simulink model "Backup"  (R2018a)
settings: Solver=VariableStepAuto  StartTime=0.0  StopTime=3  RelTol=1e-3
libraries: powerlib x15, simulink x4, rectifier_leg x3, inverter_leg x3, powerlib_meascontrol x1
settings Model: Creator=elasfory  LastModifiedBy=AL-MOSTAFA

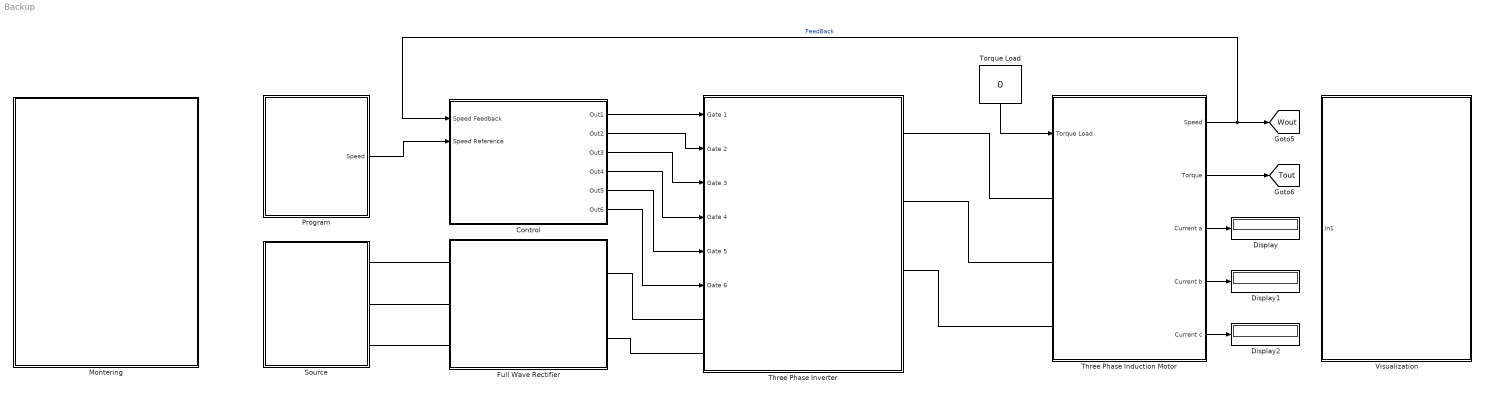
== system Backup ==
  Control : Subsystem
  Display : Display
  Display1 : Display
  Display2 : Display
  Full Wave Rectifier : Subsystem
  Montering : Subsystem
  Program : Subsystem
  Source : Subsystem
  Three Phase Induction Motor : Subsystem
  Three Phase Inverter : Subsystem
  Torque Load : Constant  Value=0
  Visualization : Subsystem
  tag scope: Tout=global, Wout=global
  wires:
  Control/6(Out6) -> Three Phase Inverter/6(Gate 6)
  Control/5(Out5) -> Three Phase Inverter/5(Gate 5)
  Control/4(Out4) -> Three Phase Inverter/4(Gate 4)
  Control/3(Out3) -> Three Phase Inverter/3(Gate 3)
  Control/2(Out2) -> Three Phase Inverter/2(Gate 2)
  Control/1(Out1) -> Three Phase Inverter/1(Gate 1)
  Three Phase Induction Motor/1(Speed) -> Control/1(Speed Feedback), [Wout]  "FeedBack"
  Three Phase Induction Motor/2(Torque) -> [Tout]
  Torque Load/1 -> Three Phase Induction Motor/1(Torque Load)
  Program/1(Speed) -> Control/2(Speed Reference)
  Three Phase Induction Motor/3(Current a) -> Display/1
  Three Phase Induction Motor/4(Current b) -> Display1/1
  Three Phase Induction Motor/5(Current c) -> Display2/1
  connections:
  Three Phase Inverter/LConn1 -- Full Wave Rectifier/RConn1
  Full Wave Rectifier/RConn2 -- Three Phase Inverter/LConn2
  Source/RConn1 -- Full Wave Rectifier/LConn1
  Source/RConn2 -- Full Wave Rectifier/LConn2
  Source/RConn3 -- Full Wave Rectifier/LConn3
  Three Phase Inverter/RConn1 -- Three Phase Induction Motor/LConn1
  Three Phase Inverter/RConn2 -- Three Phase Induction Motor/LConn2
  Three Phase Inverter/RConn3 -- Three Phase Induction Motor/LConn3

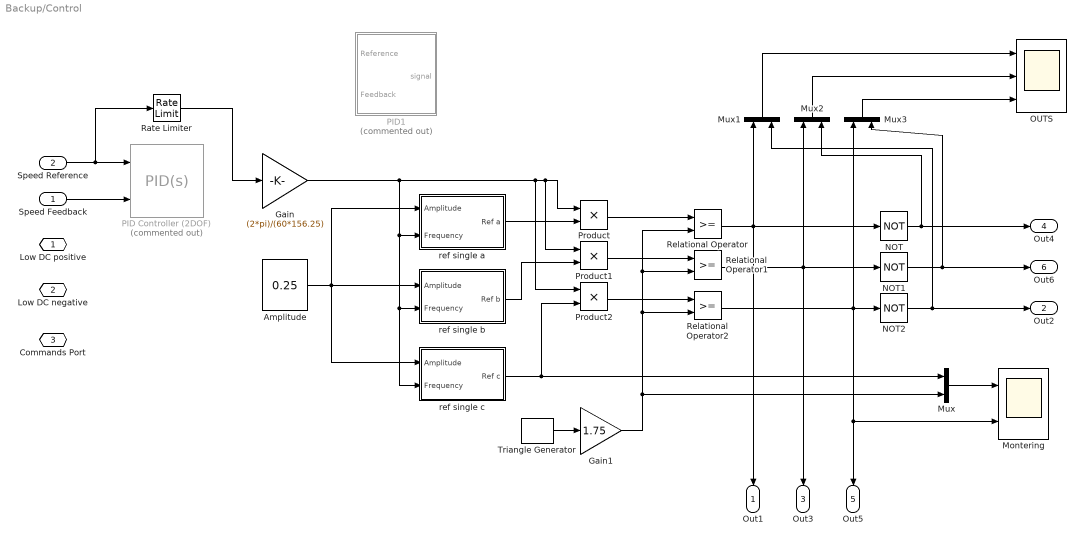
== system Backup/Control ==
  Speed Feedback : Inport
  Speed Reference : Inport  Port=2
  Amplitude : Constant  Value=0.25
  Gain : Gain  Gain=(2*pi)/(60*156.25)
  Gain1 : Gain  Gain=1.75
  Montering : Scope  NumInputPorts=2
  Mux{,1..3} (4 alike) : Mux  Inputs=2
  NOT : Logic  Operator=NOT  IconShape=distinctive  AllPortsSameDT=off  OutDataTypeStr=boolean
  NOT1 : Logic  Operator=NOT  IconShape=distinctive  AllPortsSameDT=off  OutDataTypeStr=boolean
  NOT2 : Logic  Operator=NOT  IconShape=distinctive  AllPortsSameDT=off  OutDataTypeStr=boolean
  OUTS : Scope  NumInputPorts=3
  PID Controller (2DOF) : simulink/Continuous/PID Controller (2DOF)  Commented=on  Controller=PID  TimeDomain=Continuous-time  SampleTime=-1  IntegratorMethod=Forward Euler  FilterMethod=Forward Euler  Form=Parallel  UseFilter=on  ControllerParametersSource=internal  P=1  I=0.1  D=0  N=100  b=1  c=1  InitialConditionSource=internal  InitialConditionForIntegrator=0  InitialConditionForFilter=0  ExternalReset=none  LimitOutput=off  UpperSaturationLimit=inf  LowerSaturationLimit=-inf  LinearizeAsGain=on  AntiWindupMode=none  Kb=1  TrackingMode=off  Kt=1  PParamMin=[]  PParamMax=[]  IParamMin=[]  IParamMax=[]  DParamMin=[]  DParamMax=[]  NParamMin=[]  NParamMax=[]  bParamMin=[]  bParamMax=[]  cParamMin=[]  cParamMax=[]  KbParamMin=[]  KbParamMax=[]  KtParamMin=[]  KtParamMax=[]  POutMin=[]  POutMax=[]  IOutMin=[]  IOutMax=[]  DOutMin=[]  DOutMax=[]  NOutMin=[]  NOutMax=[]  bOutMin=[]  bOutMax=[]  cOutMin=[]  cOutMax=[]  KbOutMin=[]  KbOutMax=[]  KtOutMin=[]  KtOutMax=[]  IntegratorOutMin=[]  IntegratorOutMax=[]  FilterOutMin=[]  FilterOutMax=[]  SumOutMin=[]  SumOutMax=[]  Sum1OutMin=[]  Sum1OutMax=[]  Sum2OutMin=[]  Sum2OutMax=[]  Sum3OutMin=[]  Sum3OutMax=[]  SumI1OutMin=[]  SumI1OutMax=[]  SumI2OutMin=[]  SumI2OutMax=[]  SumI3OutMin=[]  SumI3OutMax=[]  SumDOutMin=[]  SumDOutMax=[]  SaturationOutMin=[]  SaturationOutMax=[]  IntegratorContinuousStateAttributes=''  IntegratorStateMustResolveToSignalObject=off  IntegratorRTWStateStorageClass=Auto  FilterContinuousStateAttributes=''  FilterStateMustResolveToSignalObject=off  FilterRTWStateStorageClass=Auto  DifferentiatorICPrevScaledInput=0  DifferentiatorOutMin=[]  DifferentiatorOutMax=[]  FilterDiffOutCoefMin=[]  FilterDiffOutCoefMax=[]  SumDenOutMin=[]  SumDenOutMax=[]  SumNumOutMin=[]  SumNumOutMax=[]  ReciprocalOutMin=[]  ReciprocalOutMax=[]  DivideOutMin=[]  DivideOutMax=[]  TunerSelectOption=Transfer Function Based (PID Tuner App)
  PID1 : Subsystem  Commented=on
  Product : Product
  Product1 : Product
  Product2 : Product
  Rate Limiter : RateLimiter  RisingSlewLimit=100  SampleTimeMode=inherited
  Relational Operator : RelationalOperator  OutDataTypeStr=boolean  RndMeth=Simplest
  Relational Operator1 : RelationalOperator  OutDataTypeStr=boolean  RndMeth=Simplest
  Relational Operator2 : RelationalOperator  OutDataTypeStr=boolean  RndMeth=Simplest
  Triangle Generator : powerlib_meascontrol/Pulse & Signal Generators/Triangle Generator  Freq=1e4  Phase=90  Ts=0
  ref single a : Subsystem
  ref single b : Subsystem
  ref single c : Subsystem
  Low DC positive : PMIOPort  Side=Left
  Low DC negative : PMIOPort  Port=2  Side=Left
  Commands Port : PMIOPort  Port=3  Side=Left
  Out1 : Outport
  Out2 : Outport  Port=2
  Out3 : Outport  Port=3
  Out4 : Outport  Port=4
  Out5 : Outport  Port=5
  Out6 : Outport  Port=6
  wires:
  Relational Operator/1 -> Mux1/1, NOT/1, Out1/1
  Relational Operator1/1 -> Mux2/1, Out3/1, NOT1/1
  Relational Operator2/1 -> Mux3/1, Montering/2, Out5/1, NOT2/1
  Triangle Generator/1 -> Gain1/1
  NOT/1 -> Mux2/2, Out4/1
  NOT1/1 -> Mux3/2, Out6/1
  NOT2/1 -> Mux1/2, Out2/1
  ref single a/1(Ref a) -> Product/2
  ref single b/1(Ref b) -> Product1/2
  ref single c/1(Ref c) -> Product2/2, Mux/1
  Gain/1 -> ref single c/2(Frequency), ref single b/2(Frequency), ref single a/2(Frequency), Product2/1, Product/1, Product1/1
  Product/1 -> Relational Operator/1
  Product1/1 -> Relational Operator1/1
  Product2/1 -> Relational Operator2/1
  Amplitude/1 -> ref single a/1(Amplitude), ref single c/1(Amplitude), ref single b/1(Amplitude)
  Gain1/1 -> Relational Operator2/2, Relational Operator1/2, Relational Operator/2, Mux/2
  Mux/1 -> Montering/1
  Speed Reference/1 -> Rate Limiter/1, PID Controller (2DOF)/1
  Speed Feedback/1 -> PID Controller (2DOF)/2
  Rate Limiter/1 -> Gain/1
  Mux1/1 -> OUTS/1
  Mux2/1 -> OUTS/2
  Mux3/1 -> OUTS/3

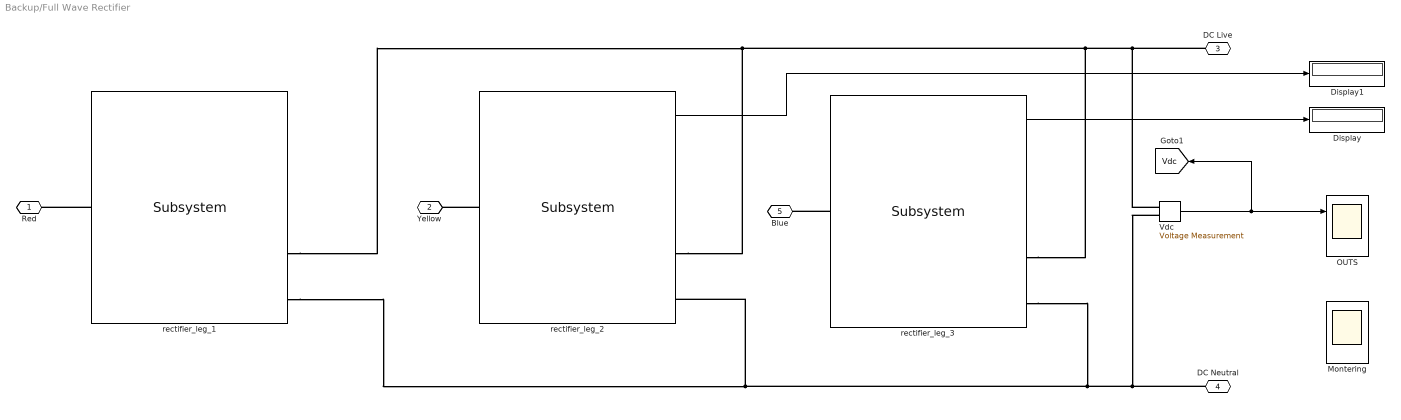
== system Backup/Full Wave Rectifier ==
  Display : Display
  Display1 : Display
  Montering : Scope  NumInputPorts=4
  OUTS : Scope  NumInputPorts=2
  Vdc : powerlib/Measurements/Voltage Measurement  PhasorSimulation=off  OutputType=Complex  PSBequivalent=0
  rectifier_leg_1 : rectifier_leg/Subsystem
  rectifier_leg_2 : rectifier_leg/Subsystem
  rectifier_leg_3 : rectifier_leg/Subsystem
  Red : PMIOPort  Side=Left
  Yellow : PMIOPort  Port=2  Side=Left
  DC Live : PMIOPort  Port=3  Side=Right
  DC Neutral : PMIOPort  Port=4  Side=Right
  Blue : PMIOPort  Port=5  Side=Left
  tag scope: Vdc=global
  wires:
  Vdc/1 -> [Vdc], OUTS/1
  rectifier_leg_3/1 -> Display/1
  rectifier_leg_2/1 -> Display1/1
  connections:
  DC Live/RConn1 -- Vdc/LConn1 -- rectifier_leg_1/RConn1 -- rectifier_leg_2/RConn1 -- rectifier_leg_3/RConn1
  rectifier_leg_1/LConn1 -- Red/RConn1
  rectifier_leg_2/LConn1 -- Yellow/RConn1
  rectifier_leg_3/LConn1 -- Blue/RConn1
  rectifier_leg_3/RConn2 -- DC Neutral/RConn1 -- Vdc/LConn2 -- rectifier_leg_2/RConn2 -- rectifier_leg_1/RConn2

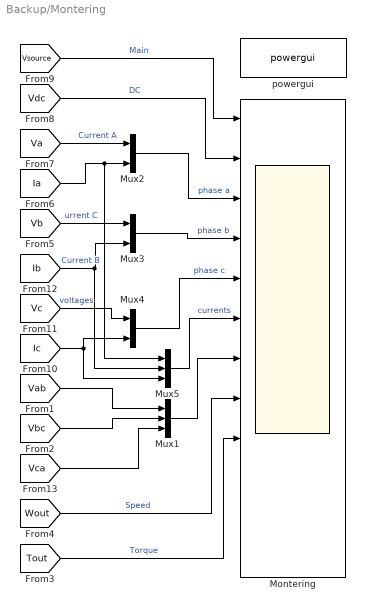
== system Backup/Montering ==
  Montering : Scope  NumInputPorts=12
  Mux1 : Mux  Inputs=3
  Mux2 : Mux  Inputs=2
  Mux3 : Mux  Inputs=2
  Mux4 : Mux  Inputs=2
  Mux5 : Mux  Inputs=3
  powergui : powerlib/powergui  Priority=1  SimulationMode=Continuous  SampleTime=50e-6  frequency=60  Iterations=50  frequencyindice=0  Pbase=100e6  ErrMax=1e-4  UnitsV=kV  UnitsW=MW  buscounter=0  FunctionMessages=off  echomessages=off  EnableUseOfTLC=off  CurrentSourceSwitches=off  DisableSnubberDevices=off  DisableRonSwitches=off  DisableVfSwitches=off  DisplayEquations=off  SolverType=Tustin/Backward Euler (TBE)  Interpol=off  ExternalGateDelay=off  methode=off  Ts=100  x0status=blocks  SPID=on  SwTol=0  HookPort=off  RestoreLinks=warning  ResistiveCurrentMeasurement=off  Frange=[0:2:500]  Ylog=off  Xlog=on  ShowGrid=off  save=off  variable=ZData  structure=0  ZoomFFT=off  StartTime=0.0  cycles=1  DisplayStyle=1  fundamental=60  FreqAxis=off  MaxFrequency=1000  frequencyindicesteady=1  RmsSteady=1  display=off
  wires:
  Mux5/1 -> Montering/6  "currents"
  [Vc] -> Mux4/1  "voltages"
  [Tout] -> Montering/9  "Torque"
  [Wout] -> Montering/8  "Speed"
  [Ic] -> Mux5/3, Mux4/2
  [Vdc] -> Montering/2  "DC"
  [Vb] -> Mux3/1  "urrent C"
  [Vbc] -> Mux1/2
  Mux1/1 -> Montering/7
  [Va] -> Mux2/1  "Current A"
  [Ib] -> Mux5/2, Mux3/2
  [Vca] -> Mux1/3
  [Vab] -> Mux1/1
  Mux3/1 -> Montering/4  "phase b"
  Mux2/1 -> Montering/3  "phase a"
  Mux4/1 -> Montering/5  "phase c"
  [Ia] -> Mux5/1, Mux2/2  "Current B"
  [Vsource] -> Montering/1  "Main"

== system Backup/Program ==
  RPM : Constant  Value=1400
  Speed : Outport
  wires:
  RPM/1 -> Speed/1

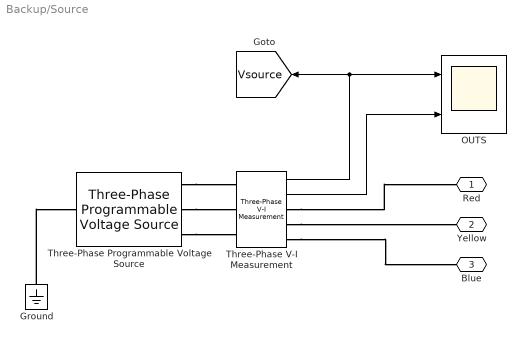
== system Backup/Source ==
  Ground : powerlib/Elements/Ground  LConnTagsString=a
  OUTS : Scope  NumInputPorts=2
  Three-Phase Programmable Voltage Source : powerlib/Electrical Sources/Three-Phase Programmable Voltage Source  PositiveSequence="[380  0 50]"  VariationEntity=None  VariationType=Table of time-amplitude pairs  VariationTypeAlt=Step  VariationStep=0.5  VariationRate=10  VariationMagnitude=0.3  VariationFrequency=2  VariationTiming=[1 2]  VariationPhaseA=off  Amplitudes=[1 0.8 1.2 1.0]  TimeValues=[0 0.1 0.15 0.2]  HarmonicGeneration=off  HarmonicA=[3 0.2 -25 0]  HarmonicB=[2 0.15 35 2]  Timing="[0.05  3]"  BusType=swing  Pref=0  Qref=0  Qmin=-inf  Qmax=inf
  Three-Phase V-I Measurement : powerlib/Measurements/Three-Phase V-I Measurement  VoltageMeasurement=phase-to-ground  SetLabelV=off  LabelV=Vabc  Vpu=off  VpuLL=off  CurrentMeasurement=yes  SetLabelI=off  LabelI=Iabc  Ipu=off  Pbase=100e6  Vbase=500e3  OutputType=Complex  PhasorSimulation=off  PSBequivalent=0
  Red : PMIOPort  Side=Right
  Yellow : PMIOPort  Port=2  Side=Right
  Blue : PMIOPort  Port=3  Side=Right
  tag scope: Vsource=global
  wires:
  Three-Phase V-I Measurement/1 -> [Vsource], OUTS/1
  Three-Phase V-I Measurement/2 -> OUTS/2
  connections:
  Three-Phase V-I Measurement/RConn3 -- Blue/RConn1
  Three-Phase V-I Measurement/RConn1 -- Red/RConn1
  Three-Phase V-I Measurement/RConn2 -- Yellow/RConn1
  Three-Phase Programmable Voltage Source/RConn1 -- Three-Phase V-I Measurement/LConn1
  Three-Phase Programmable Voltage Source/RConn2 -- Three-Phase V-I Measurement/LConn2
  Three-Phase Programmable Voltage Source/RConn3 -- Three-Phase V-I Measurement/LConn3
  Ground/LConn1 -- Three-Phase Programmable Voltage Source/LConn1

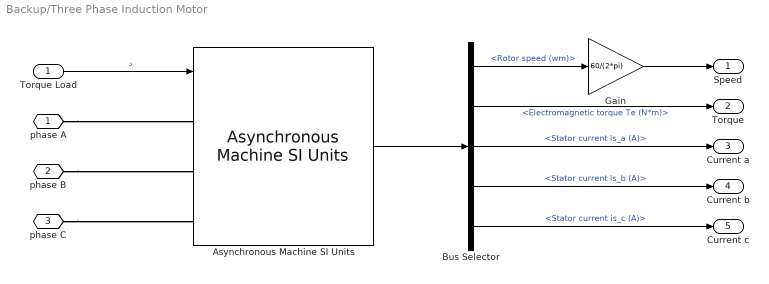
== system Backup/Three Phase Induction Motor ==
  Torque Load : Inport
  Asynchronous Machine SI Units : powerlib/Machines/Asynchronous Machine SI Units  RotorType=Squirrel-cage  PresetModel="15:  5.4 HP (4KW)   400 V  50Hz 1430 RPM"  MechanicalLoad=Torque Tm  ShowDetailedParameters=on  ReferenceFrame=Stationary  Units=SI  MeasurementBus=off  NominalParameters=[4000 400 50]  Stator=[1.405 0.005839]  Rotor=[1.395 0.005839]  Cage1=[0.4155 0.002066]  Cage2=[0.4168 0.0003495]  Lm=0.1722  Mechanical=[0.0131 0.002985 2]  PolePairs=2  InitialConditions=[1 0 0 0 0 0 0 0]  SimulateSaturation=off  Saturation=[14.03593122, 27.81365428, 53.79336849, 72.68890987, 97.98006896, 148.6815601, 215.7428561, 302.9841135, 428.7778367 ; 230, 322, 414, 460, 506, 552, 598, 644, 690]  LoadFlowParameters=1492000  TsPowergui=0  TsBlock=-1  IterativeModel=Trapezoidal non iterative  IterativeDiscreteModel=Trapezoidal non iterative  Pmec=1.492e+006
  Bus Selector : BusSelector  OutputSignals=Mechanical.Rotor speed (wm),Mechanical.Electromagnetic torque Te (N*m),Stator measurements.Stator current is_a (A),Stator measurements.Stator current is_b (A),Stator measurements.Stator current is_c (A)
  Gain : Gain  Gain=60/(2*pi)
  phase A : PMIOPort  Side=Left
  phase B : PMIOPort  Port=2  Side=Left
  phase C : PMIOPort  Port=3  Side=Left
  Speed : Outport
  Torque : Outport  Port=2
  Current a : Outport  Port=3
  Current b : Outport  Port=4
  Current c : Outport  Port=5
  wires:
  Asynchronous Machine SI Units/1 -> Bus Selector/1
  Bus Selector/2 -> Torque/1  "<Electromagnetic torque Te (N*m)>"
  Torque Load/1 -> Asynchronous Machine SI Units/1  "د"
  Bus Selector/3 -> Current a/1  "<Stator current is_a (A)>"
  Bus Selector/4 -> Current b/1  "<Stator current is_b (A)>"
  Bus Selector/5 -> Current c/1  "<Stator current is_c (A)>"
  Bus Selector/1 -> Gain/1  "<Rotor speed (wm)>"
  Gain/1 -> Speed/1
  connections:
  phase B/RConn1 -- Asynchronous Machine SI Units/LConn2
  phase A/RConn1 -- Asynchronous Machine SI Units/LConn1
  phase C/RConn1 -- Asynchronous Machine SI Units/LConn3

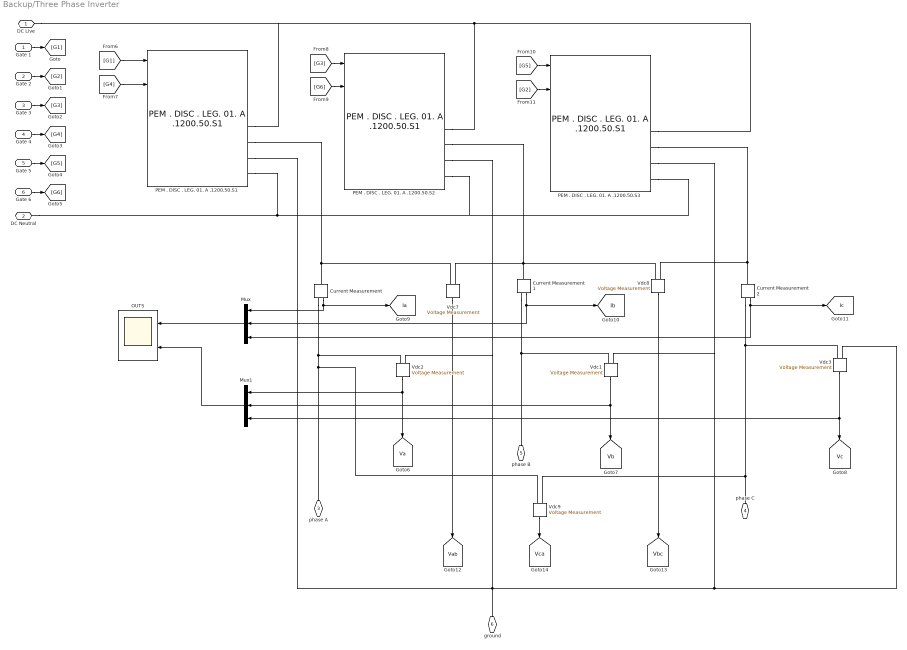
== system Backup/Three Phase Inverter ==
  Gate 1 : Inport
  Gate 2 : Inport  Port=2
  Gate 3 : Inport  Port=3
  Gate 4 : Inport  Port=4
  Gate 5 : Inport  Port=5
  Gate 6 : Inport  Port=6
  Current Measurement : powerlib/Measurements/Current Measurement  PhasorSimulation=off  OutputType=Complex  PSBequivalent=0
  Current Measurement1 : powerlib/Measurements/Current Measurement  PhasorSimulation=off  OutputType=Complex  PSBequivalent=0
  Current Measurement2 : powerlib/Measurements/Current Measurement  PhasorSimulation=off  OutputType=Complex  PSBequivalent=0
  Mux : Mux  Inputs=3
  Mux1 : Mux  Inputs=3
  OUTS : Scope  NumInputPorts=2
  PEM . DISC . LEG. 01. A .1200.50.S1 : inverter_leg/PEM . DISC . LEG. 01. A .1200.50.S1
  PEM . DISC . LEG. 01. A .1200.50.S2 : inverter_leg/PEM . DISC . LEG. 01. A .1200.50.S1
  PEM . DISC . LEG. 01. A .1200.50.S3 : inverter_leg/PEM . DISC . LEG. 01. A .1200.50.S1
  Vdc{1..3,7..9} (6 alike) : powerlib/Measurements/Voltage Measurement  PhasorSimulation=off  OutputType=Complex  PSBequivalent=0
  DC Live : PMIOPort  Side=Left
  DC Neutral : PMIOPort  Port=2  Side=Left
  phase A : PMIOPort  Port=3  Side=Right
  phase C : PMIOPort  Port=4  Side=Right
  phase B : PMIOPort  Port=5  Side=Right
  ground : PMIOPort  Port=6  Side=Right
  tag scope: Ia=global, Ib=global, Ic=global, Va=global, Vab=global, Vb=global, Vbc=global, Vc=global, Vca=global
  wires:
  Gate 1/1 -> [G1]
  Gate 2/1 -> [G2]
  Gate 3/1 -> [G3]
  Gate 4/1 -> [G4]
  Gate 5/1 -> [G5]
  Gate 6/1 -> [G6]
  [G4] -> PEM . DISC . LEG. 01. A .1200.50.S1/2
  [G1] -> PEM . DISC . LEG. 01. A .1200.50.S1/1
  [G6] -> PEM . DISC . LEG. 01. A .1200.50.S2/2
  [G3] -> PEM . DISC . LEG. 01. A .1200.50.S2/1
  [G5] -> PEM . DISC . LEG. 01. A .1200.50.S3/1
  [G2] -> PEM . DISC . LEG. 01. A .1200.50.S3/2
  Current Measurement/1 -> [Ia], Mux/1
  Current Measurement1/1 -> Mux/2, [Ib]
  Current Measurement2/1 -> Mux/3, [Ic]
  Vdc2/1 -> [Va], Mux1/1
  Vdc1/1 -> Mux1/2, [Vb]
  Vdc3/1 -> Mux1/3, [Vc]
  Vdc9/1 -> [Vca]
  Vdc7/1 -> [Vab]
  Vdc8/1 -> [Vbc]
  Mux/1 -> OUTS/1
  Mux1/1 -> OUTS/2
  connections:
  PEM . DISC . LEG. 01. A .1200.50.S1/RConn1 -- DC Live/RConn1 -- PEM . DISC . LEG. 01. A .1200.50.S3/RConn1 -- PEM . DISC . LEG. 01. A .1200.50.S2/RConn1
  PEM . DISC . LEG. 01. A .1200.50.S3/RConn4 -- PEM . DISC . LEG. 01. A .1200.50.S2/RConn4 -- PEM . DISC . LEG. 01. A .1200.50.S1/RConn4 -- DC Neutral/RConn1
  ground/RConn1 -- PEM . DISC . LEG. 01. A .1200.50.S1/RConn3 -- PEM . DISC . LEG. 01. A .1200.50.S3/RConn3 -- Vdc1/LConn2 -- Vdc3/LConn2 -- PEM . DISC . LEG. 01. A .1200.50.S2/RConn3 -- Vdc2/LConn2
  Current Measurement/LConn1 -- PEM . DISC . LEG. 01. A .1200.50.S1/RConn2 -- Vdc7/LConn1
  Current Measurement/RConn1 -- Vdc2/LConn1 -- Vdc9/LConn2 -- phase A/RConn1
  Current Measurement1/RConn1 -- Vdc1/LConn1 -- phase B/RConn1
  Current Measurement1/LConn1 -- PEM . DISC . LEG. 01. A .1200.50.S2/RConn2 -- Vdc8/LConn1 -- Vdc7/LConn2
  Current Measurement2/RConn1 -- Vdc3/LConn1 -- Vdc9/LConn1 -- phase C/RConn1
  Current Measurement2/LConn1 -- PEM . DISC . LEG. 01. A .1200.50.S3/RConn2 -- Vdc8/LConn2

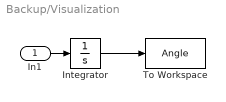
== system Backup/Visualization ==
  In1 : Inport
  Integrator : Integrator
  To Workspace : ToWorkspace  VariableName=Angle  SaveFormat=Timeseries  SampleTime=0.001
      settings: MaxDataPoints=10
  wires:
  Integrator/1 -> To Workspace/1
  In1/1 -> Integrator/1

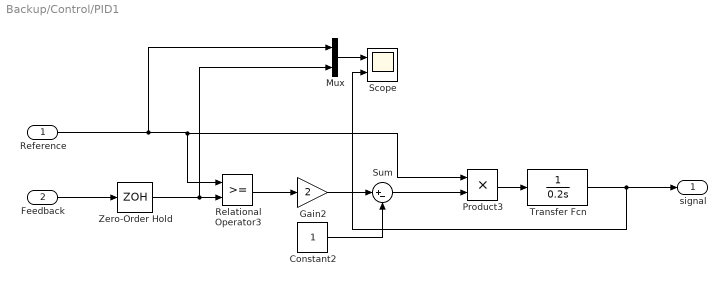
== system Backup/Control/PID1 ==
  Reference : Inport
  Feedback : Inport  Port=2
  Constant2 : Constant
  Gain2 : Gain  Gain=2
  Mux : Mux  Inputs=2
  Product3 : Product
  Relational Operator3 : RelationalOperator  OutDataTypeStr=boolean  RndMeth=Simplest
  Scope : Scope  NumInputPorts=2
  Sum : Sum  Inputs=|+-
  Transfer Fcn : TransferFcn  Denominator=[0.2 0]
  Zero-Order Hold : ZeroOrderHold  SampleTime=1e-2
  signal : Outport
  wires:
  Zero-Order Hold/1 -> Mux/2, Relational Operator3/2
  Relational Operator3/1 -> Gain2/1
  Constant2/1 -> Sum/2
  Sum/1 -> Product3/2
  Gain2/1 -> Sum/1
  Product3/1 -> Transfer Fcn/1
  Reference/1 -> Mux/1, Product3/1, Relational Operator3/1
  Transfer Fcn/1 -> Scope/2, signal/1
  Mux/1 -> Scope/1
  Feedback/1 -> Zero-Order Hold/1

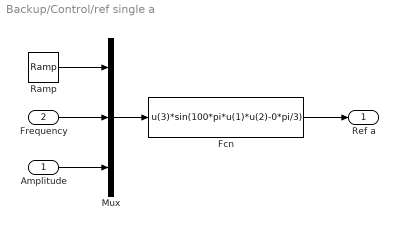
== system Backup/Control/ref single a ==
  Amplitude : Inport
  Frequency : Inport  Port=2
  Fcn : Fcn  Expr=u(3)*sin(100*pi*u(1)*u(2)-0*pi/3)
  Mux : Mux  Inputs=3
  Ramp : simulink/Sources/Ramp  slope=1  start=0  InitialOutput=0
  Ref a : Outport
  wires:
  Mux/1 -> Fcn/1
  Frequency/1 -> Mux/2
  Ramp/1 -> Mux/1
  Fcn/1 -> Ref a/1
  Amplitude/1 -> Mux/3

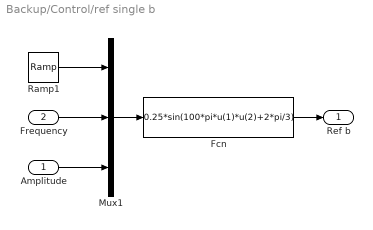
== system Backup/Control/ref single b ==
  Amplitude : Inport
  Frequency : Inport  Port=2
  Fcn : Fcn  Expr=0.25*sin(100*pi*u(1)*u(2)+2*pi/3)
  Mux1 : Mux  Inputs=3
  Ramp1 : simulink/Sources/Ramp  slope=1  start=0  InitialOutput=0
  Ref b : Outport
  wires:
  Fcn/1 -> Ref b/1
  Ramp1/1 -> Mux1/1
  Frequency/1 -> Mux1/2
  Mux1/1 -> Fcn/1
  Amplitude/1 -> Mux1/3

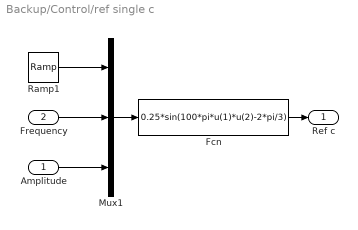
== system Backup/Control/ref single c ==
  Amplitude : Inport
  Frequency : Inport  Port=2
  Fcn : Fcn  Expr=0.25*sin(100*pi*u(1)*u(2)-2*pi/3)
  Mux1 : Mux  Inputs=3
  Ramp1 : simulink/Sources/Ramp  slope=1  start=0  InitialOutput=0
  Ref c : Outport
  wires:
  Fcn/1 -> Ref c/1
  Amplitude/1 -> Mux1/3
  Mux1/1 -> Fcn/1
  Frequency/1 -> Mux1/2
  Ramp1/1 -> Mux1/1
